simulink model "Duke_Simulink_13a"  (R2013a)
settings: Solver=FixedStepDiscrete  StartTime=0  StopTime=tempoSimulacao  FixedStep=1  RelTol=1e-3
values from neighbouring files (symbols this model uses):
  Ajustes_Inicial = dadosNumeroConstantes(linha)    [read_parametros_v2.m]
  aliquotaIR = dadosNumeroConstantes(linha)    [read_parametros_v2.m]
  CaixaInicial = dadosNumeroConstantes(linha)    [read_parametros_v2.m]
  Capital_Social_Inicial = CapitalSocial(1,2:end)    [Duke_main_v2.m]
  CFURH = dadosNumeroConstantes(linha)*TAR    [read_parametros_v2.m]
  contribuicaoCCEE = dadosNumeroConstantes(linha)    [read_parametros_v2.m]
  deducaoP_D = dadosNumeroConstantes(linha)    [read_parametros_v2.m]
  den_Ajustes = [1 zeros(1,PeriodoDepreciacao_Ajustes)]    [gera_Input_modelo.m]
  den_CustoAnual = [1 zeros(1,PeriodoCustoAnual-1)]    [gera_Input_modelo.m]
  den_CustoSemestral = [1 zeros(1,PeriodoCustoSemestral-1)]    [gera_Input_modelo.m]
  den_PPE_Edificacoes = [1 zeros(1,PPE_Periodo_Edificacoes)]    [gera_Input_modelo.m]
  den_PPE_Maquinas = [1 zeros(1,PPE_Periodo_Maquinas)]    [gera_Input_modelo.m]
  den_PPE_Moveis = [1 zeros(1,PPE_Periodo_Moveis)]    [gera_Input_modelo.m]
  den_PPE_Reservatorio = [1 zeros(1,PPE_Periodo_Reservatorio)]    [gera_Input_modelo.m]
  den_PPE_Veiculos = [1 zeros(1,PPE_Periodo_Veiculos)]    [gera_Input_modelo.m]
  DividaInicial = MtM_Total_Dividas(1,2:end)    [Duke_main_v2.m]
  Dividendos_A_Pagar_Inicial = dadosNumeroConstantes(linha)    [read_parametros_v2.m]
  garantiaFisica = dadosNumeroConstantes(linha)    [read_parametros_v2.m]
  IC_DividendosAPagarInicial = [repmat(vetor_DividendosAPagarInicial(1),numRealidades,1); zeros(realidadesPorSimulacao-numRealidades,1)]    [gera_Input_modelo.m]
  inicializa_JSCP = zeros(realidadesPorSimulacao,mes_JSCP)    [Duke_main_v2.m]
  IR_diferido_acumulado_inicial = dadosNumeroConstantes(linha)    [read_parametros_v2.m]
  JSCP_A_Pagar_Inicial = dadosNumeroConstantes(linha)    [read_parametros_v2.m]
  JSCP_ParcialPeriodo = dadosNumeroConstantes(linha)    [read_parametros_v2.m]
  JSCP_RetidoInicial = 0    [Duke_main_v2.m]
  Limite_Reserva_Lucros = dadosNumeroConstantes(linha)    [read_parametros_v2.m]
  Limite_Reserva_Lucros_Capital = dadosNumeroConstantes(linha)    [read_parametros_v2.m]
  LucroParcialPeriodo = dadosNumeroConstantes(linha)    [read_parametros_v2.m]
  LucroRetidoInicial = dadosNumeroConstantes(linha)    [read_parametros_v2.m]
  mes_DataInicial = month(DataInicial)    [Duke_main_v2.m]
  mes_JSCP = dadosNumeroConstantes(linha)    [read_parametros_v2.m]
  num_Ajustes = [0 ones(1,PeriodoDepreciacao_Ajustes)]*(1/PeriodoDepreciacao_Ajustes)    [gera_Input_modelo.m]
  num_CustoAnual = ones(1,PeriodoCustoAnual)*(1/PeriodoCustoAnual)    [gera_Input_modelo.m]
  num_CustoSemestral = ones(1,PeriodoCustoSemestral)*(1/PeriodoCustoSemestral)    [gera_Input_modelo.m]
  num_PPE_Edificacoes = [0 ones(1,PPE_Periodo_Edificacoes)]*(1/PPE_Periodo_Edificacoes)    [gera_Input_modelo.m]
  num_PPE_Maquinas = [0 ones(1,PPE_Periodo_Maquinas)]*(1/PPE_Periodo_Maquinas)    [gera_Input_modelo.m]
  num_PPE_Moveis = [0 ones(1,PPE_Periodo_Moveis)]*(1/PPE_Periodo_Moveis)    [gera_Input_modelo.m]
  num_PPE_Reservatorio = [0 ones(1,PPE_Periodo_Reservatorio)]*(1/PPE_Periodo_Reservatorio)    [gera_Input_modelo.m]
  num_PPE_Veiculos = [0 ones(1,PPE_Periodo_Veiculos)]*(1/PPE_Periodo_Veiculos)    [gera_Input_modelo.m]
  Outros_Passivos = dadosNumeroConstantes(linha)    [read_parametros_v2.m]
  periodoDividendos = dadosNumeroConstantes(linha)    [read_parametros_v2.m]
  periodoDividendos_delay = periodoDividendos    [Duke_main_v2.m]
  PeriodoIR_diferido = 12    [Duke_main_v2.m]
  PeriodoJSCP = 12    [Duke_main_v2.m]
  PIS_COFINS_Cumulativo = PIS + COFINS    [read_parametros_v2.m]
  PPE_Inicial_Edificacoes = dadosNumeroConstantes(linha)    [read_parametros_v2.m]
  PPE_Inicial_Maquinas = dadosNumeroConstantes(linha)    [read_parametros_v2.m]
  PPE_Inicial_Moveis = dadosNumeroConstantes(linha)    [read_parametros_v2.m]
  PPE_Inicial_Reservatorio = dadosNumeroConstantes(linha)    [read_parametros_v2.m]
  PPE_Inicial_Terreno = dadosNumeroConstantes(linha)    [read_parametros_v2.m]
  PPE_Inicial_Veiculos = dadosNumeroConstantes(linha)    [read_parametros_v2.m]
  refInd = (1-TEIFref)*(1-TEIPref)    [read_parametros_v2.m]
  Reserva_Capital_Inicial = dadosNumeroConstantes(linha)    [read_parametros_v2.m]
  Reserva_Lucros_Inicial = dadosNumeroConstantes(linha)    [read_parametros_v2.m]
  Taxa_Anual_Reserva = dadosNumeroConstantes(linha)    [read_parametros_v2.m]
  Taxa_diferimento = dadosNumeroConstantes(linha)    [read_parametros_v2.m]
  taxaMinorityInterest = dadosNumeroConstantes(linha)    [read_parametros_v2.m]
  TEIFa = dadosNumeroConstantes(linha)    [read_parametros_v2.m]
  TEIP = dadosNumeroConstantes(linha)    [read_parametros_v2.m]
  tempoSimulacao = 180    [Duke_main_v2.m]
  TEO = dadosNumeroConstantes(linha)    [read_parametros_v2.m]
  vetor_DividendosAPagarInicial = [repmat(vetor_DividendosAPagarInicial,numRealidades,1); zeros(realidadesPorSimulacao-numRealidades,periodoDividendos)]    [gera_Input_modelo.m]
  vetor_JSCP_APagarInicial = [repmat(vetor_JSCP_APagarInicial,numRealidades,1); zeros(realidadesPorSimulacao-numRealidades,PeriodoJSCP)]    [gera_Input_modelo.m]
undefined symbols (not defined in the file or in its folder): aDeducaoICMS, DiaPgtDespesasAdm, DiscIntNeverNeededParam, dts, IC_JSCP_APagarInicial, juros_ContasAPagar, juros_ContasAReceber, Media_DeprPPE, mediaADeducaoICMS, mediaADeducaoPISCOFINS, mediaRuidoGeracao, mediaTEIFa, mediaTEIP, Parametros, Periodo_Mes, PPE_Inicial, r, ruidoGeracaoSeed, Seed_DeprPPE, seedADeducaoICMS, seedADeducaoPISCOFINS, TEIFaSeed, TEIPSeed, Var_DeprPPE, varianciaADeducaoICMS, varianciaADeducaoPISCOFINS, varianciaRuidoGeracao, varianciaTEIFa, varianciaTEIP
libraries: simulink x22, dspsrcs4 x12
(part 1 of 2)
settings Model: TunableVars=Ajustes_Inicial,CFURH,CaixaInicial,Capital_Social_Inicial,DividaInicial,IC_DividendosAPagarInicial,IR_diferido_acumulado_inicial,JSCP_ParcialPeriodo,JSCP_RetidoInicial,Limite_Reserva_Lucros,Limite_Reserva_Lucros_Capital,LucroParcialPeriodo,LucroRetidoInicial,Outros_Passivos,PIS_COFINS_Cumulativo,PPE_Inicial_Edificacoes,PPE_Inicial_Maquinas,PPE_Inicial_Moveis,PPE_Inicial_Reservatorio,PPE_Inicial_Terreno,PPE_Inicial_Veiculos,PeriodoIR_diferido,PeriodoJSCP,Reserva_Capital_Inicial,Reserva_Lucros_Inicial,TEIFa,TEIP,TEO,TFSEE,Taxa_Anual_Reserva,Taxa_diferimento,aliquotaIR,contribuicaoCCEE,deducaoP_D,den_Ajustes,den_PPE_Edificacoes,den_PPE_Maquinas,den_PPE_Moveis,den_PPE_Reservatorio,den_PPE_Veiculos,den_Premio,garantiaFisica,inicializa_JSCP,mes_DataInicial,mes_JSCP,num_Ajustes,num_PPE_Edificacoes,num_PPE_Maquinas,num_PPE_Moveis,num_PPE_Reservatorio,num_PPE_Veiculos,num_Premio,periodoDividendos,periodoDividendos_delay,refInd,taxaMinorityInterest,vetor_DividendosAPagarInicial,vetor_JSCP_APagarInicial  TunableVarsStorageClass=Auto,Auto,Auto,Auto,Auto,Auto,Auto,Auto,Auto,Auto,Auto,Auto,Auto,Auto,Auto,Auto,Auto,Auto,Auto,Auto,Auto,Auto,Auto,Auto,Auto,Auto,Auto,Auto,Auto,Auto,Auto,Auto,Auto,Auto,Auto,Auto,Auto,Auto,Auto,Auto,Auto,Auto,Auto,Auto,Auto,Auto,Auto,Auto,Auto,Auto,Auto,Auto,Auto,Auto,Auto,Auto,Auto,Auto  TunableVarsTypeQualifier=,,,,,,,,,,,,,,,,,,,,,,,,,,,,,,,,,,,,,,,,,,,,,,,,,,,,,,,,,  Creator=sergio.junior  LastModifiedBy=Felipe
settings DataIOCC: ExternalInput=Input  LoadExternalInput=on  SaveFormat=StructureWithTime
settings OptimizationCC: InlineParams=on  ExpressionDepthLimit=2147483647
settings DebuggingCC: MultiTaskDSMMsg=warning  MultiTaskCondExecSysMsg=none  MultiTaskRateTransMsg=warning
settings HardwareCC: TargetIntDivRoundTo=Zero  TargetEndianess=LittleEndian  TargetHWDeviceType=MATLAB Host  ProdEqTarget=off
settings SFSimCC: SimParseCustomCode=off
settings RTWCC: SystemTargetFile=rsim.tlc  TemplateMakefile=rsim_default_tmf  Description=Rapid Simulation Target  ProcessScript=rsim_make_rtw_hook  IncludeERTFirstTime=on  RTWCompilerOptimization=On
settings RSimTargetCC: CodeReplacementLibrary=C89/C90 (ANSI)  ERTMultiwordTypeDef=System defined  ERTMultiwordLength=256  IsPILTarget=off  LogVarNameModifier=none  EnableShiftOperators=on  RSIM_SOLVER_SELECTION=UseSolverModule

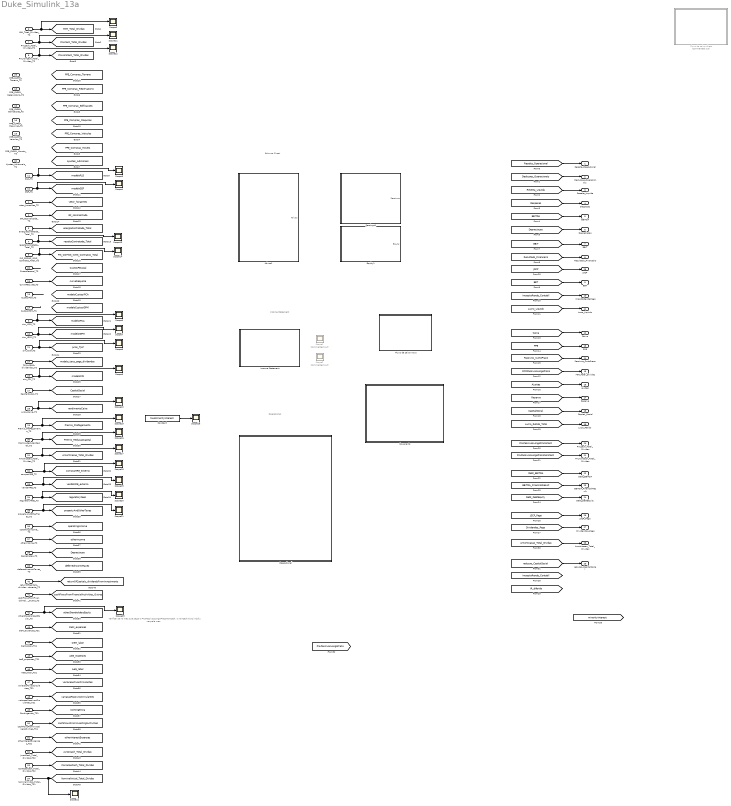
== system Duke_Simulink_13a ==
  note: Operacional
  note: Income Statement
  note: Balance Sheet
  note: Verificar se no mes que paga o PnLPassivosLongoPrazoNonCash, o nonCash é oq incidiu naquele mes
  vetor_horasMes_TS : Inport
  GF_sazonalizada_TS : Inport  Port=2
  energiaContratada_Total_TS : Inport  Port=3
  receitaContratada_Total_TS : Inport  Port=4  PortDimensions=realidadesPorSimulacao
  PIS_COFINS_ICMS_Contratos_Total_TS : Inport  Port=5  PortDimensions=realidadesPorSimulacao
  MtM_Total_Dividas_TS : Inport  Port=6  PortDimensions=realidadesPorSimulacao
  PnLCash_Total_Dividas_TS : Inport  Port=7  PortDimensions=realidadesPorSimulacao
  PnLnonCash_Total_Dividas_TS : Inport  Port=8  PortDimensions=realidadesPorSimulacao
  sim_IPCA_TS : Inport  Port=9  PortDimensions=realidadesPorSimulacao
  sim_IGPM_TS : Inport  Port=10  PortDimensions=realidadesPorSimulacao
  PLD_TS : Inport  Port=11  PortDimensions=realidadesPorSimulacao
  GSF_TS : Inport  Port=12  PortDimensions=realidadesPorSimulacao
  CustosIPCA_TS : Inport  Port=13
  CustosIGPM_TS : Inport  Port=14
  PPE_CAPEX_Edificacoes_TS : Inport  Port=15
  PPE_CAPEX_Maquinas_TS : Inport  Port=16
  PPE_CAPEX_Moveis_TS : Inport  Port=17
  PPE_CAPEX_Reservatorio_TS : Inport  Port=18
  PPE_CAPEX_Veiculos_TS : Inport  Port=19
  Ajustes_Adicionais_TS : Inport  Port=20
  sim_TJLP_TS : Inport  Port=21  PortDimensions=realidadesPorSimulacao
  CustosPessoal_TS : Inport  Port=22
  CurvaReajuste_TS : Inport  Port=23
  taxa_paga_dividendos_TS : Inport  Port=24
  sim_CDI_TS : Inport  Port=25  PortDimensions=realidadesPorSimulacao
  PPE_CAPEX_Terreno_TS : Inport  Port=26
  CapitalSocial_TS : Inport  Port=27
  juros_Caixa_TS : Inport  Port=28  PortDimensions=realidadesPorSimulacao
  Premio_PrePagamento_TS : Inport  Port=29  PortDimensions=realidadesPorSimulacao
  Premio_ReducaoCapital_TS : Inport  Port=30  PortDimensions=realidadesPorSimulacao
  Amortizacao_Total_Dividas_TS : Inport  Port=31  PortDimensions=realidadesPorSimulacao
  compraMRE_TS : Inport  Port=32
  vendaMRE_TS : Inport  Port=33
  regulatoryFees_TS : Inport  Port=34
  propertyAndOtherTaxes_TS : Inport  Port=35
  operatingIncome_TS : Inport  Port=36
  otherIncome_TS : Inport  Port=37
  depreciacao_TS : Inport  Port=38
  deferredIncomeTaxes_TS : Inport  Port=39
  returnOfCapitals_dividendsFromInvestments_TS : Inport  Port=40
  cashFlowsFromFinancialActivities_Outros_TS : Inport  Port=41
  otherShareholdersEquity_TS : Inport  Port=42
  OeM_expenses_TS1 : Inport  Port=43
  OeM_labor_TS1 : Inport  Port=44
  AeG_expenses_TS1 : Inport  Port=45
  AeG_labor_TS1 : Inport  Port=46
  variacaoAtivosCirculantes_TS1 : Inport  Port=47
  variacaoPassivosCirculantes_TS1 : Inport  Port=48
  Contingencia_TS1 : Inport  Port=49
  cashFlowsFromInvestinglActivities_TS1 : Inport  Port=50
  otherInterestExpenses_TS2 : Inport  Port=51
  JurosCash_Total_Dividas_TS2 : Inport  Port=52  PortDimensions=realidadesPorSimulacao
  CorrecaoCash_Total_Dividas_TS2 : Inport  Port=53  PortDimensions=realidadesPorSimulacao
  NominalInicial_Total_Dividas_TS1 : Inport  Port=54
  Ativos1 : Subsystem
  Constant : Constant  Value=taxaMinorityInterest
  Covenants : Subsystem
  Equity1 : Subsystem
  Fluxo de caixa direto : Subsystem  Commented=on
  Fluxo de caixa novo : Subsystem
  Income Statement : Subsystem
  Operacional : Subsystem
  Passivos1 : Subsystem
  Scope1 : Scope  Commented=on
      settings: TimeRange=500  YMin=-50000  YMax=450000  SaveName=ScopeData10
  Scope{3..22,25..26} (22 alike) : Scope
      Scope10 settings: YMin=0  YMax=65000  SaveName=ScopeData132
      Scope11 settings: YMin=0  YMax=65000  SaveName=ScopeData133
      Scope12 settings: YMin=0  YMax=65000  SaveName=ScopeData134
      Scope13 settings: YMin=0  YMax=65000  SaveName=ScopeData135
      Scope14 settings: YMin=0  YMax=65000  SaveName=ScopeData136
      Scope15 settings: YMin=0  YMax=65000  SaveName=ScopeData163
      Scope16 settings: YMin=0  YMax=65000  SaveName=ScopeData164
      Scope17 settings: YMin=0  YMax=65000  SaveName=ScopeData167
      Scope18 settings: YMin=0  YMax=65000  SaveName=ScopeData169
      Scope19 settings: YMin=0  YMax=65000  SaveName=ScopeData170
      Scope20 settings: YMin=0  YMax=65000  SaveName=ScopeData171
      Scope21 settings: YMin=0  YMax=65000  SaveName=ScopeData172
      Scope22 settings: YMin=0  YMax=65000  SaveName=ScopeData89
      Scope25 settings: YMin=0  YMax=65000  SaveName=ScopeData176
      Scope26 settings: YMin=0  YMax=65000  SaveName=ScopeData177
      Scope3 settings: YMin=0  YMax=65000  SaveName=ScopeData126
      Scope4 settings: YMin=0  YMax=65000  SaveName=ScopeData127
      Scope5 settings: YMin=0  YMax=65000  SaveName=ScopeData128
      Scope6 settings: YMin=0  YMax=65000  SaveName=ScopeData118
      Scope7 settings: YMin=0  YMax=65000  SaveName=ScopeData129
      Scope8 settings: YMin=0  YMax=65000  SaveName=ScopeData130
      Scope9 settings: YMin=0  YMax=65000  SaveName=ScopeData131
  Scope2 : Scope  Commented=on
      settings: TimeRange=500  YMin=-50000  YMax=450000  SaveName=ScopeData11
  Receita_Operacional : Outport
  Deducoes_Operacionais : Outport  Port=2
  Receita_Liquida : Outport  Port=3
  Despesas : Outport  Port=4
  EBITDA : Outport  Port=5
  Depreciacao : Outport  Port=6
  EBIT : Outport  Port=7
  Resultado_Financeiro : Outport  Port=8
  EBT : Outport  Port=9
  ImpostoRendaPago : Outport  Port=10
  Lucro_Liquido : Outport  Port=11
  Caixa : Outport  Port=12
  PPE : Outport  Port=13
  Passivos_CurtoPrazo : Outport  Port=14
  MtM_Total_Dividas : Outport  Port=15
  Ajustes : Outport  Port=16
  Reserva : Outport  Port=17
  Capital_Social : Outport  Port=18
  Lucro_Retido : Outport  Port=19
  PnLCash_Total_Dividas : Outport  Port=20
  PnLnonCash_Total_Dividas : Outport  Port=21
  Debt_EBITDA : Outport  Port=22
  EBITDA_FinancialResult : Outport  Port=23
  Debt_DebtEquity : Outport  Port=24
  JSCP : Outport  Port=25
  JSCP_Pago : Outport  Port=26
  Dividendos_Pago : Outport  Port=27
  Amortizacao_Total_Dividas : Outport  Port=28
  reducao_CapitalSocial : Outport  Port=29
  tag scope: AeG_expenses=global, AeG_labor=global, Ajustes_Adicionais=global, Amortizacao_Total_Dividas=global, CapitalSocial=global, Contingencia=global, CorrecaoCash_Total_Dividas=global, CustosPessoal=global, Depreciacao=global, GF_sazonalizada=global, JurosCash_Total_Dividas=global, MtM_Total_Dividas=global, NominalInicial_Total_Dividas=global, OeM_expenses=global, OeM_labor=global, PIS_COFINS_ICMS_Contratos_Total=global, PPE_Compras_Edificacoes=global, PPE_Compras_Maquinas=global, PPE_Compras_Moveis=global, PPE_Compras_Reservatorio=global, PPE_Compras_Terreno=global, PPE_Compras_Veiculos=global, PnLCash_Total_Dividas=global, PnLnonCash_Total_Dividas=global, Premio_PrePagamento=global, Premio_ReducaoCapital=global, cashFlowsFromFinancialActivities_Outros=global, cashFlowsFromInvestinglActivities=global, compraMRE_externo=global, curvaReajuste=global, deferredIncomeTaxes=global, energiaContratada_Total=global, juros_TJLP=global, modeloCDI=global, modeloCustosIGPM=global, modeloCustosIPCA=global, modeloGSF=global, modeloIGPM=global, modeloIPCA=global, modeloPLD=global, modelo_taxa_paga_dividendos=global, operatingIncome=global, otherIncome=global, otherInterestExpenses=global, otherShareholdersEquity=global, propertyAndOtherTaxes=global, receitaContratada_Total=global, regulatoryFees=global, rendimentoCaixa=global, returnOfCapitals_dividendsFromInvestments=global, variacaoAtivosCirculantes=global, variacaoPassivosCirculantes=global, vendaMRE_externo=global, vetor_horasMes=global
  wires:
  [Receita_Operacional] -> Receita_Operacional/1
  [Deducoes_Operacionais] -> Deducoes_Operacionais/1
  [Receita_Liquida] -> Receita_Liquida/1
  [Despesas] -> Despesas/1
  [EBITDA] -> EBITDA/1
  [Depreciacao] -> Depreciacao/1
  [EBIT] -> EBIT/1
  [Resultado_Financeiro] -> Resultado_Financeiro/1
  [EBT] -> EBT/1
  [ImpostoRenda_Contabil] -> ImpostoRendaPago/1
  [Lucro_Liquido] -> Lucro_Liquido/1
  [Caixa] -> Caixa/1
  [PPE] -> PPE/1
  [Passivos_CurtoPrazo] -> Passivos_CurtoPrazo/1
  [MtMPassivosLongoPrazo] -> MtM_Total_Dividas/1
  [Ajustes] -> Ajustes/1
  [Reserva] -> Reserva/1
  [CapitalSocial] -> Capital_Social/1
  [Lucro_Retido_Total] -> Lucro_Retido/1
  [PnLPassivosLongoPrazoCash] -> PnLCash_Total_Dividas/1
  [PnLPassivosLongoPrazoNonCash] -> PnLnonCash_Total_Dividas/1
  [Debt_EBITDA] -> Debt_EBITDA/1
  [EBITDA_FinancialResult] -> EBITDA_FinancialResult/1
  [Debt_DebtEquity] -> Debt_DebtEquity/1
  MtM_Total_Dividas_TS/1 -> Scope6/1, [MtM_Total_Dividas]
  PnLCash_Total_Dividas_TS/1 -> Scope11/1, [PnLCash_Total_Dividas]
  PnLnonCash_Total_Dividas_TS/1 -> Scope12/1, [PnLnonCash_Total_Dividas]
  ? -> [PPE_Compras_Reservatorio]
  ? -> [PPE_Compras_Edificacoes]
  ? -> [PPE_Compras_Maquinas]
  ? -> [PPE_Compras_Veiculos]
  ? -> [PPE_Compras_Moveis]
  ? -> [Ajustes_Adicionais]
  PLD_TS/1 -> Scope3/1, [modeloPLD]
  GSF_TS/1 -> Scope4/1, [modeloGSF]
  vetor_horasMes_TS/1 -> [vetor_horasMes]
  GF_sazonalizada_TS/1 -> [GF_sazonalizada]
  energiaContratada_Total_TS/1 -> [energiaContratada_Total]
  receitaContratada_Total_TS/1 -> Scope13/1, [receitaContratada_Total]
  PIS_COFINS_ICMS_Contratos_Total_TS/1 -> Scope14/1, [PIS_COFINS_ICMS_Contratos_Total]
  CustosPessoal_TS/1 -> ?
  CurvaReajuste_TS/1 -> [curvaReajuste]
  CustosIPCA_TS/1 -> ?
  CustosIGPM_TS/1 -> ?
  sim_IPCA_TS/1 -> Scope5/1, [modeloIPCA]
  sim_IGPM_TS/1 -> Scope7/1, [modeloIGPM]
  sim_TJLP_TS/1 -> Scope8/1, [juros_TJLP]
  [JSCP] -> JSCP/1
  taxa_paga_dividendos_TS/1 -> [modelo_taxa_paga_dividendos]
  sim_CDI_TS/1 -> Scope9/1, [modeloCDI]
  ? -> [PPE_Compras_Terreno]
  CapitalSocial_TS/1 -> [CapitalSocial]
  juros_Caixa_TS/1 -> Scope10/1, [rendimentoCaixa]
  [JSCP_Pago] -> JSCP_Pago/1
  [Dividendos_Pago] -> Dividendos_Pago/1
  Premio_PrePagamento_TS/1 -> [Premio_PrePagamento], Scope15/1
  Premio_ReducaoCapital_TS/1 -> [Premio_ReducaoCapital], Scope16/1
  Amortizacao_Total_Dividas_TS/1 -> Scope17/1, [Amortizacao_Total_Dividas]
  [Amortizacao_Total_Dividas] -> Amortizacao_Total_Dividas/1
  [reducao_CapitalSocial] -> reducao_CapitalSocial/1
  compraMRE_TS/1 -> Scope18/1, [compraMRE_externo]
  vendaMRE_TS/1 -> Scope19/1, [vendaMRE_externo]
  regulatoryFees_TS/1 -> Scope20/1, [regulatoryFees]
  propertyAndOtherTaxes_TS/1 -> Scope21/1, [propertyAndOtherTaxes]
  operatingIncome_TS/1 -> [operatingIncome]
  otherIncome_TS/1 -> [otherIncome]
  depreciacao_TS/1 -> [Depreciacao]
  deferredIncomeTaxes_TS/1 -> [deferredIncomeTaxes]
  returnOfCapitals_dividendsFromInvestments_TS/1 -> [returnOfCapitals_dividendsFromInvestments]
  cashFlowsFromFinancialActivities_Outros_TS/1 -> [cashFlowsFromFinancialActivities_Outros]
  otherShareholdersEquity_TS/1 -> Scope25/1, [otherShareholdersEquity]
  Constant/1 -> Scope26/1
  OeM_expenses_TS1/1 -> [OeM_expenses]
  OeM_labor_TS1/1 -> [OeM_labor]
  AeG_expenses_TS1/1 -> [AeG_expenses]
  AeG_labor_TS1/1 -> [AeG_labor]
  variacaoAtivosCirculantes_TS1/1 -> [variacaoAtivosCirculantes]
  variacaoPassivosCirculantes_TS1/1 -> [variacaoPassivosCirculantes]
  Contingencia_TS1/1 -> [Contingencia]
  cashFlowsFromInvestinglActivities_TS1/1 -> [cashFlowsFromInvestinglActivities]
  otherInterestExpenses_TS2/1 -> [otherInterestExpenses]
  JurosCash_Total_Dividas_TS2/1 -> [JurosCash_Total_Dividas]
  CorrecaoCash_Total_Dividas_TS2/1 -> [CorrecaoCash_Total_Dividas]
  NominalInicial_Total_Dividas_TS1/1 -> Scope22/1, [NominalInicial_Total_Dividas]

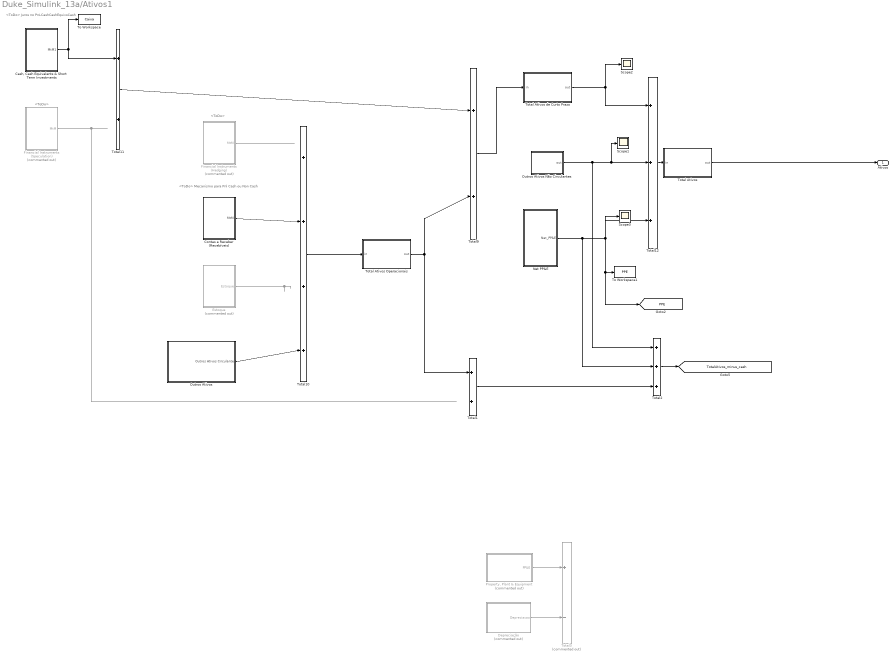
== system Duke_Simulink_13a/Ativos1 ==
  note: <ToDo>
      | Mecanismo para
      | Pnl Cash ou Non Cash
  note: <ToDo>
  note: <ToDo>
      | Juros no
      | PnLCashCashEquivsCash
  note: <ToDo>
  "Cash, Cash Equivalents & Short Term Investments" : Subsystem
  Contas a Receber (Recebíveis) : Subsystem
  Depreciação : Subsystem  Commented=on
  Estoque : Subsystem  Commented=on
  Financial Instruments (Hedging) : Subsystem  Commented=on
  Financial Instruments (Speculation) : Subsystem  Commented=on
  Net PP&E : Subsystem
  Outros Ativos : Subsystem
  Outros Ativos Não Circulantes : Subsystem
  "Property, Plant & Equipment" : Subsystem  Commented=on
  Scope1 : Scope
      settings: SaveName=ScopeData73
  Scope2 : Scope
      settings: SaveName=ScopeData74
  Scope3 : Scope
      settings: SaveName=ScopeData72
  To Workspace : ToWorkspace  VariableName=Caixa  SampleTime=-1  SaveFormat=Timeseries
  To Workspace1 : ToWorkspace  VariableName=PPE  SampleTime=-1  SaveFormat=Timeseries
  Total Ativos : Subsystem
  Total Ativos Operacionais : Subsystem
  Total Ativos de Curto Prazo : Subsystem
  Total1 : Sum
  Total10 : Sum  Inputs=+|+|+|+
  Total11 : Sum  Inputs=+|+
  Total12 : Sum  Inputs=+||+||+
  Total2 : Sum  Inputs=+++
  Total3 : Sum  Commented=on  Inputs=+-
  Total9 : Sum  Inputs=+||+
  "Ativos    " : Outport
  tag scope: PPE=global, TotalAtivos_minus_cash=global
  wires:
  Estoque/1(Estoque) -> ?
  Financial Instruments (Speculation)/1(MtM) -> ?
  Financial Instruments (Hedging)/1(MtM) -> ?
  Total11/1 -> Total9/1
  Total10/1 -> Total Ativos Operacionais/1(in)
  Total Ativos Operacionais/1(out) -> Total9/2, Total1/1
  Total9/1 -> Total Ativos de Curto Prazo/1(in)
  Total12/1 -> Total Ativos/1(in)
  Total Ativos de Curto Prazo/1(out) -> Scope2/1, Total12/1
  "Cash, Cash Equivalents & Short Term Investments"/1(MtM1) -> To Workspace/1, Total11/1
  Total1/1 -> Total2/3
  Total2/1 -> [TotalAtivos_minus_cash]
  "Property, Plant & Equipment"/1(PP&E) -> Total3/1
  Outros Ativos Não Circulantes/1(out) -> Total2/1, Scope1/1, Total12/2
  Net PP&E/1(Net_PP&E) -> Total2/2, Total12/3, Scope3/1, To Workspace1/1, [PPE]
  Depreciação/1(Depreciacao) -> Total3/2
  Outros Ativos/1(Outros Ativos Circulantes) -> Total10/4
  Contas a Receber (Recebíveis)/1(MtM) -> Total10/2
  Total Ativos/1(out) -> "Ativos    "/1

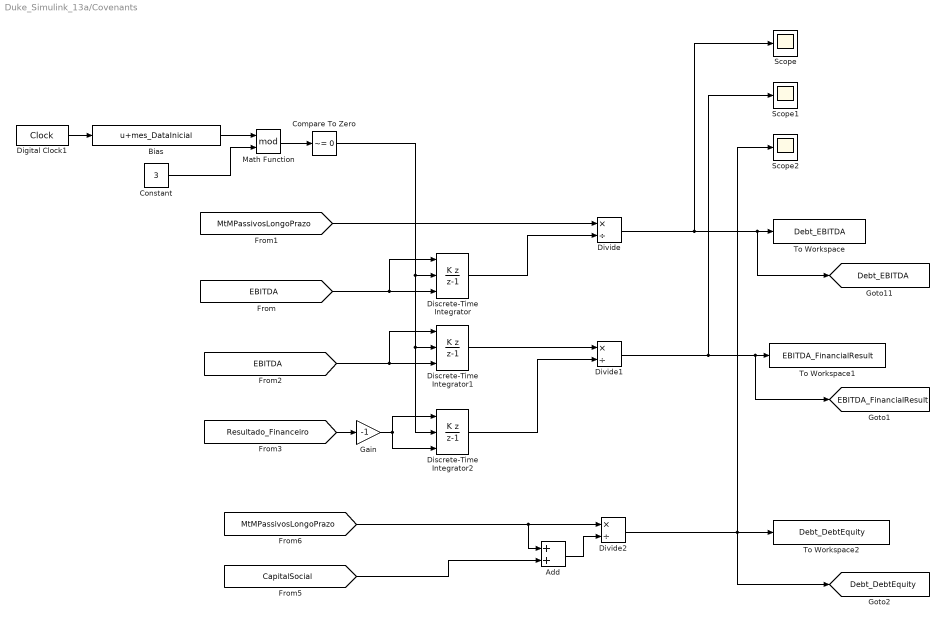
== system Duke_Simulink_13a/Covenants ==
  Add : Sum
  Bias : Bias  Bias=mes_DataInicial
  Compare To Zero : simulink/Logic and Bit Operations/Compare To Zero  relop=~=  OutDataTypeStr=boolean
  Constant : Constant  Value=3
  Digital Clock1 : DigitalClock
  Discrete-Time Integrator : DiscreteIntegrator  IntegratorMethod=Accumulation: Backward Euler  ExternalReset=rising  InitialConditionSource=external  ICPrevOutput=DiscIntNeverNeededParam  ICPrevScaledInput=DiscIntNeverNeededParam
  Discrete-Time Integrator1 : DiscreteIntegrator  IntegratorMethod=Accumulation: Backward Euler  ExternalReset=rising  InitialConditionSource=external  ICPrevOutput=DiscIntNeverNeededParam  ICPrevScaledInput=DiscIntNeverNeededParam
  Discrete-Time Integrator2 : DiscreteIntegrator  IntegratorMethod=Accumulation: Backward Euler  ExternalReset=rising  InitialConditionSource=external  ICPrevOutput=DiscIntNeverNeededParam  ICPrevScaledInput=DiscIntNeverNeededParam
  Divide : Product  Inputs=*/  SampleTime=1
  Divide1 : Product  Inputs=*/  SampleTime=1
  Divide2 : Product  Inputs=*/  SampleTime=1
  Gain : Gain  Gain=-1
  Math Function : Math  Operator=mod  SaturateOnIntegerOverflow=on
  Scope : Scope
      settings: SaveName=ScopeData47
  Scope1 : Scope
      settings: SaveName=ScopeData48
  Scope2 : Scope
      settings: SaveName=ScopeData49
  To Workspace : ToWorkspace  VariableName=Debt_EBITDA  SampleTime=1  SaveFormat=Timeseries
  To Workspace1 : ToWorkspace  VariableName=EBITDA_FinancialResult  SampleTime=1  SaveFormat=Timeseries
  To Workspace2 : ToWorkspace  VariableName=Debt_DebtEquity  SampleTime=1  SaveFormat=Timeseries
  tag scope: Debt_DebtEquity=global, Debt_EBITDA=global, EBITDA_FinancialResult=global
  wires:
  [EBITDA] -> Discrete-Time Integrator/1, Discrete-Time Integrator/3
  Divide/1 -> [Debt_EBITDA], To Workspace/1, Scope/1
  Divide1/1 -> Scope1/1, [EBITDA_FinancialResult], To Workspace1/1
  Divide2/1 -> [Debt_DebtEquity], Scope2/1, To Workspace2/1
  Constant/1 -> Math Function/2
  Math Function/1 -> Compare To Zero/1
  Compare To Zero/1 -> Discrete-Time Integrator2/2, Discrete-Time Integrator1/2, Discrete-Time Integrator/2
  [EBITDA] -> Discrete-Time Integrator1/1, Discrete-Time Integrator1/3
  [Resultado_Financeiro] -> Gain/1
  [MtMPassivosLongoPrazo] -> Divide/1
  Discrete-Time Integrator/1 -> Divide/2
  Discrete-Time Integrator1/1 -> Divide1/1
  Discrete-Time Integrator2/1 -> Divide1/2
  [MtMPassivosLongoPrazo] -> Add/1, Divide2/1
  Gain/1 -> Discrete-Time Integrator2/1, Discrete-Time Integrator2/3
  Add/1 -> Divide2/2
  [CapitalSocial] -> Add/2
  Digital Clock1/1 -> Bias/1
  Bias/1 -> Math Function/1

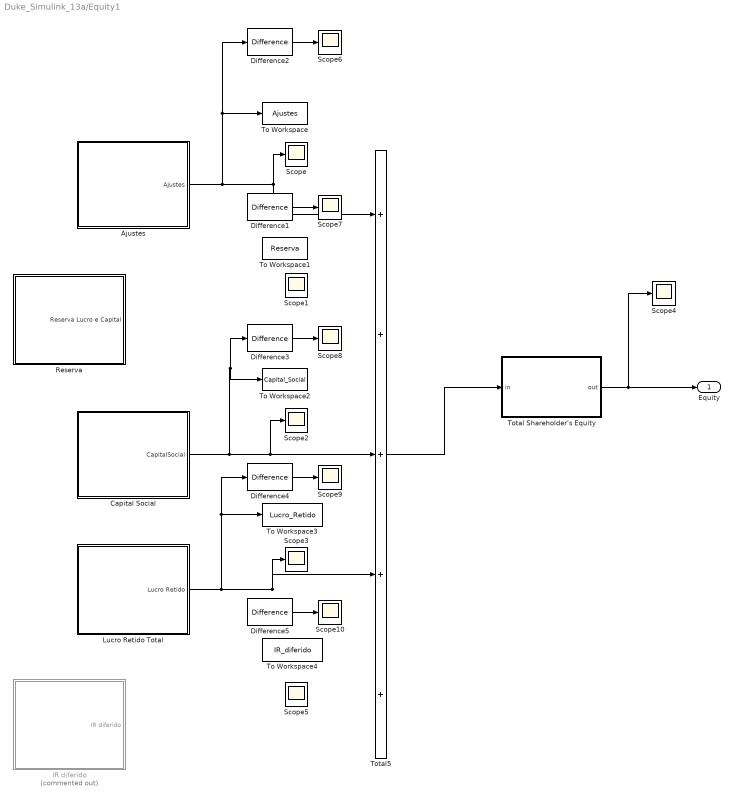
== system Duke_Simulink_13a/Equity1 ==
  Ajustes : Subsystem
  Capital Social : Subsystem
  Difference{1..5} (5 alike) : simulink/Discrete/Difference  ICPrevInput=0  InputProcessing=Inherited  OutMin=[]  OutMax=[]  OutDataType=fixdt(1, 16)  OutScaling=2^-10  DoSatur=off
  IR diferido : Subsystem  Commented=on
  Lucro Retido Total : Subsystem
  Reserva : Subsystem
  Scope{,1..10} (11 alike) : Scope
      Scope settings: SaveName=ScopeData81
      Scope1 settings: SaveName=ScopeData82
      Scope10 settings: SaveName=ScopeData153
      Scope2 settings: SaveName=ScopeData83
      Scope3 settings: SaveName=ScopeData84
      Scope4 settings: SaveName=ScopeData36
      Scope5 settings: SaveName=ScopeData119
      Scope6 settings: SaveName=ScopeData149
      Scope7 settings: SaveName=ScopeData150
      Scope8 settings: SaveName=ScopeData151
      Scope9 settings: SaveName=ScopeData152
  To Workspace : ToWorkspace  VariableName=Ajustes  SampleTime=-1  SaveFormat=Timeseries
  To Workspace1 : ToWorkspace  VariableName=Reserva  SampleTime=-1  SaveFormat=Timeseries
  To Workspace2 : ToWorkspace  VariableName=Capital_Social  SampleTime=-1  SaveFormat=Timeseries
  To Workspace3 : ToWorkspace  VariableName=Lucro_Retido  SampleTime=-1  SaveFormat=Timeseries
  To Workspace4 : ToWorkspace  VariableName=IR_diferido  SampleTime=-1  SaveFormat=Timeseries
  Total Shareholder's Equity : Subsystem
  Total5 : Sum  Inputs=+|+|+|+|+
  "Equity    " : Outport
  wires:
  Lucro Retido Total/1(Lucro Retido) -> Difference4/1, To Workspace3/1, Scope3/1, Total5/4
  Total5/1 -> Total Shareholder's Equity/1(in)
  Ajustes/1(Ajustes) -> Difference2/1, To Workspace/1, Scope/1, Total5/1
  ? -> Difference1/1, To Workspace1/1, Scope1/1, Total5/2
  Capital Social/1(CapitalSocial) -> Difference3/1, To Workspace2/1, Scope2/1, Total5/3
  Total Shareholder's Equity/1(out) -> Scope4/1, "Equity    "/1
  ? -> Total5/5, Scope5/1, Difference5/1, To Workspace4/1
  Difference2/1 -> Scope6/1
  Difference1/1 -> Scope7/1
  Difference3/1 -> Scope8/1
  Difference4/1 -> Scope9/1
  Difference5/1 -> Scope10/1

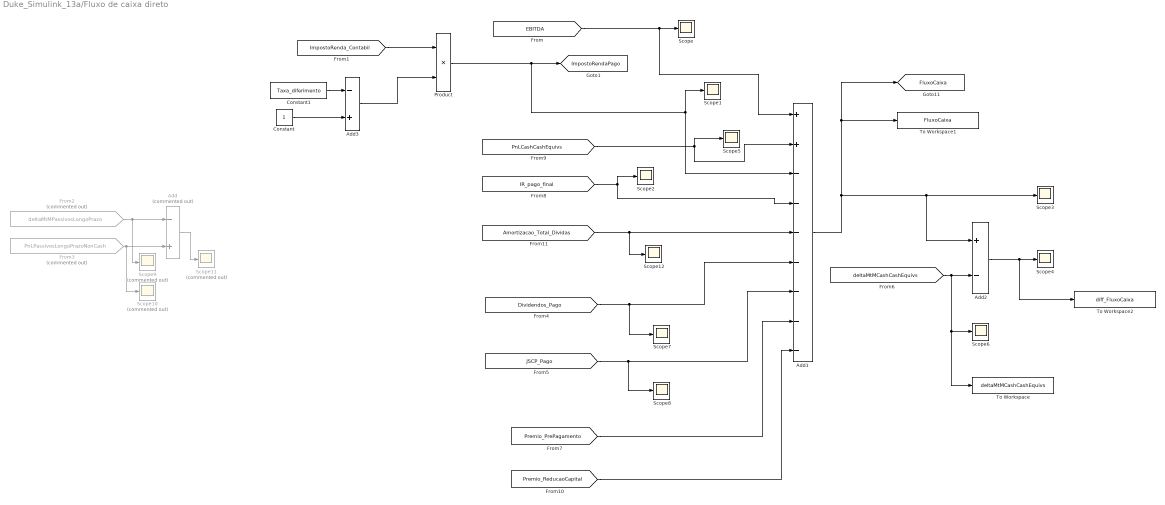
== system Duke_Simulink_13a/Fluxo de caixa direto ==
  Add : Sum  Commented=on  Inputs=-+
  Add1 : Sum  Inputs=++-------
  Add2 : Sum  Inputs=+-
  Add3 : Sum  Inputs=-+
  Constant : Constant
  Constant1 : Constant  Value=Taxa_diferimento
  From2 : From  Commented=on  GotoTag=deltaMtMPassivosLongoPrazo  TagVisibility=global
  From3 : From  Commented=on  GotoTag=PnLPassivosLongoPrazoNonCash  TagVisibility=global
  Product : Product
  Scope{,1..8,12} (10 alike) : Scope
      Scope settings: SaveName=ScopeData47
      Scope1 settings: SaveName=ScopeData48
      Scope12 settings: SaveName=ScopeData168
      Scope2 settings: SaveName=ScopeData53
      Scope3 settings: TimeRange=10  SaveName=ScopeData50
      Scope4 settings: TimeRange=450  YMin=-2e-06  YMax=2e-06  SaveName=ScopeData52
      Scope5 settings: SaveName=ScopeData125
      Scope6 settings: TimeRange=450  YMin=-15000000000  YMax=15000000000  SaveName=ScopeData66
      Scope7 settings: SaveName=ScopeData68
      Scope8 settings: SaveName=ScopeData69
  Scope10 : Scope  Commented=on
      settings: SaveName=ScopeData138
  Scope11 : Scope  Commented=on
      settings: SaveName=ScopeData139
  Scope9 : Scope  Commented=on
      settings: SaveName=ScopeData137
  To Workspace : ToWorkspace  VariableName=deltaMtMCashCashEquivs  SampleTime=-1  SaveFormat=Timeseries
  To Workspace1 : ToWorkspace  VariableName=FluxoCaixa  SampleTime=-1  SaveFormat=Timeseries
  To Workspace2 : ToWorkspace  VariableName=diff_FluxoCaixa  SampleTime=-1  SaveFormat=Timeseries
  tag scope: FluxoCaixa=global, ImpostoRendaPago=global
  wires:
  From2/1 -> Scope9/1, Add/1
  From3/1 -> Scope10/1, Add/2
  Add/1 -> Scope11/1
  Product/1 -> Add1/3, Scope1/1, [ImpostoRendaPago]
  Add2/1 -> To Workspace2/1, Scope4/1
  [deltaMtMCashCashEquivs] -> To Workspace/1, Scope6/1, Add2/2
  Add1/1 -> [FluxoCaixa], To Workspace1/1, Add2/1, Scope3/1
  [EBITDA] -> Add1/1, Scope/1
  [Dividendos_Pago] -> Add1/6, Scope7/1
  [JSCP_Pago] -> Add1/7, Scope8/1
  [ImpostoRenda_Contabil] -> Product/1
  Constant1/1 -> Add3/1
  Add3/1 -> Product/2
  Constant/1 -> Add3/2
  [IR_pago_final] -> Add1/4, Scope2/1
  [PnLCashCashEquivs] -> Scope5/1, Add1/2
  [Premio_PrePagamento] -> Add1/8
  [Premio_ReducaoCapital] -> Add1/9
  [Amortizacao_Total_Dividas] -> Scope12/1, Add1/5

== system Duke_Simulink_13a/Fluxo de caixa novo ==
  Add1 : Sum  Inputs=+-+++++++---+-+-
  Discrete-Time Integrator2 : DiscreteIntegrator  IntegratorMethod=Accumulation: Backward Euler  InitialCondition=CaixaInicial  ICPrevOutput=DiscIntNeverNeededParam  ICPrevScaledInput=DiscIntNeverNeededParam
  Scope3 : Scope
      settings: TimeRange=10  SaveName=ScopeData50
  Scope4 : Scope
      settings: TimeRange=450  YMin=-2e-06  YMax=2e-06  SaveName=ScopeData52
  tag scope: Caixa=global, cashFlow=global
  wires:
  [Lucro_Liquido] -> Add1/1
  [Depreciacao] -> Add1/2
  [minorityInterest] -> Add1/3
  [variacaoAtivosCirculantes] -> Add1/4
  [variacaoPassivosCirculantes] -> Add1/5
  [Contingencia] -> Add1/6
  [returnOfCapitals_dividendsFromInvestments] -> Add1/7
  [cashFlowsFromInvestinglActivities] -> Add1/8
  [cashFlowsFromFinancialActivities_Outros] -> Add1/9
  [JurosCash_Total_Dividas] -> Add1/11
  [CorrecaoCash_Total_Dividas] -> Add1/12
  [Amortizacao_Total_Dividas] -> Add1/10
  [NominalInicial_Total_Dividas] -> Add1/13
  ? -> Add1/14
  [PnLnonCash_Total_Dividas] -> Add1/15
  Add1/1 -> [cashFlow], Discrete-Time Integrator2/1
  Discrete-Time Integrator2/1 -> [Caixa]
  ? -> Add1/16

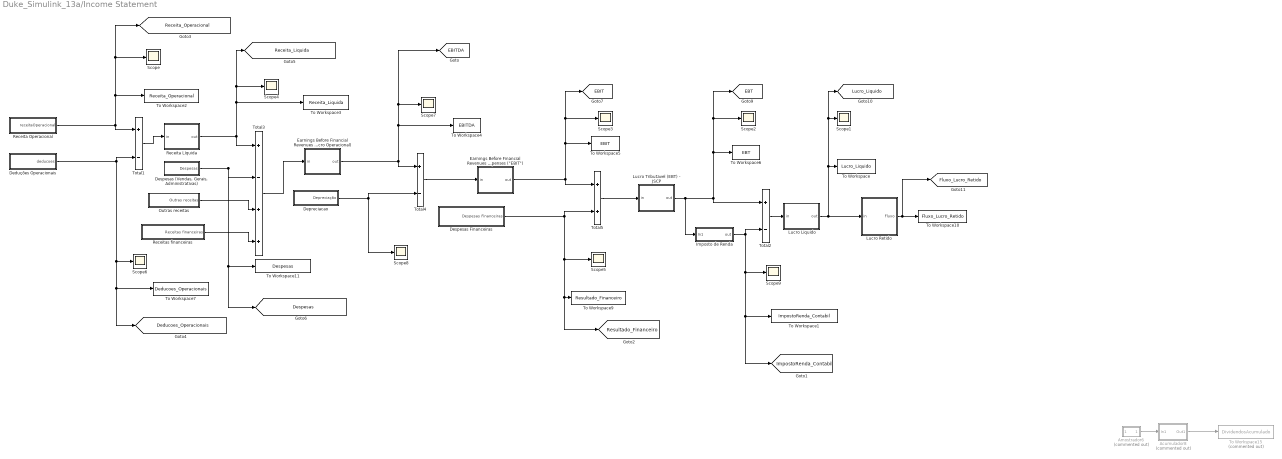
== system Duke_Simulink_13a/Income Statement ==
  Acumulador8 : Subsystem  Commented=on
  Amostrador6 : Subsystem  Commented=on
  Deduções Operacionais : Subsystem
  Depreciacao : Subsystem
  "Despesas (Vendas, Gerais, Administrativas)" : Subsystem
  Despesas Financeiras : Subsystem
  "Earnings Before Financial Revenues / Expenses, Depreciation and Amortization (\"EBITDA\") (Lucro Operacional)" : Subsystem
  "Earnings Before Financial Revenues and Expenses (\"EBIT\")" : Subsystem
  Imposto de Renda : Subsystem
  "Lucro Liquido " : Subsystem
  Lucro Retido : Subsystem
  Lucro Tributavel (EBT) - JSCP : Subsystem
  Outras receitas : Subsystem
  Receita Líquida : Subsystem
  Receita Operacional : Subsystem
  Receitas financeiras : Subsystem
  Scope{,1..9} (10 alike) : Scope
      Scope settings: SaveName=ScopeData5
      Scope1 settings: SaveName=ScopeData27
      Scope2 settings: SaveName=ScopeData28
      Scope3 settings: SaveName=ScopeData29
      Scope4 settings: SaveName=ScopeData8
      Scope5 settings: TimeRange=400  YMin=-15000000  YMax=0  SaveName=ScopeData31
      Scope6 settings: SaveName=ScopeData16
      Scope7 settings: SaveName=ScopeData15
      Scope8 settings: SaveName=ScopeData34
      Scope9 settings: SaveName=ScopeData46
  To Workspace : ToWorkspace  VariableName=Lucro_Liquido  SampleTime=-1  SaveFormat=Timeseries
  To Workspace1 : ToWorkspace  VariableName=ImpostoRenda_Contabil  SampleTime=-1  SaveFormat=Timeseries
  To Workspace10 : ToWorkspace  VariableName=Fluxo_Lucro_Retido  SampleTime=-1  SaveFormat=Timeseries
  To Workspace11 : ToWorkspace  VariableName=Despesas  SampleTime=-1  SaveFormat=Timeseries
  To Workspace15 : ToWorkspace  Commented=on  VariableName=DividendosAcumulado  SampleTime=-1  SaveFormat=Timeseries
  To Workspace2 : ToWorkspace  VariableName=Receita_Operacional  SampleTime=-1  SaveFormat=Timeseries
  To Workspace3 : ToWorkspace  VariableName=Receita_Liquida  SampleTime=-1  SaveFormat=Timeseries
  To Workspace4 : ToWorkspace  VariableName=EBITDA  SampleTime=-1  SaveFormat=Timeseries
  To Workspace5 : ToWorkspace  VariableName=EBIT  SampleTime=-1  SaveFormat=Timeseries
  To Workspace6 : ToWorkspace  VariableName=EBT  SampleTime=-1  SaveFormat=Timeseries
  To Workspace7 : ToWorkspace  VariableName=Deducoes_Operacionais  SampleTime=-1  SaveFormat=Timeseries
  To Workspace9 : ToWorkspace  VariableName=Resultado_Financeiro  SampleTime=-1  SaveFormat=Timeseries
  Total1 : Sum  Inputs=+|-
  Total2 : Sum  Inputs=+|-
  Total3 : Sum  Inputs=+|-|+|+
  Total4 : Sum  Inputs=+|-
  Total5 : Sum  Inputs=+|+
  tag scope: Deducoes_Operacionais=global, Despesas=global, EBIT=global, EBITDA=global, EBT=global, Fluxo_Lucro_Retido=global, ImpostoRenda_Contabil=global, Lucro_Liquido=global, Receita_Liquida=global, Receita_Operacional=global, Resultado_Financeiro=global
  wires:
  "Lucro Liquido "/1(out) -> Lucro Retido/1(in), [Lucro_Liquido], Scope1/1, To Workspace/1
  Acumulador8/1(Out1) -> To Workspace15/1
  Amostrador6/1(Out1) -> Acumulador8/1(In1)
  Receita Líquida/1(out) -> Total3/1, To Workspace3/1, [Receita_Liquida], Scope4/1
  "Earnings Before Financial Revenues / Expenses, Depreciation and Amortization (\"EBITDA\") (Lucro Operacional)"/1(out) -> [EBITDA], Scope7/1, To Workspace4/1, Total4/1
  Total4/1 -> "Earnings Before Financial Revenues and Expenses (\"EBIT\")"/1(in)
  "Earnings Before Financial Revenues and Expenses (\"EBIT\")"/1(out) -> To Workspace5/1, [EBIT], Scope3/1, Total5/1
  Total5/1 -> Lucro Tributavel (EBT) - JSCP/1(in)
  Lucro Tributavel (EBT) - JSCP/1(out) -> To Workspace6/1, [EBT], Scope2/1, Total2/1, Imposto de Renda/1(In1)
  Imposto de Renda/1(out) -> [ImpostoRenda_Contabil], To Workspace1/1, Scope9/1, Total2/2
  Total2/1 -> "Lucro Liquido "/1(in)
  Total1/1 -> Receita Líquida/1(in)
  Receita Operacional/1(receitaOperacional) -> To Workspace2/1, [Receita_Operacional], Scope/1, Total1/1
  Deduções Operacionais/1(deducoes) -> Scope6/1, [Deducoes_Operacionais], To Workspace7/1, Total1/2
  Depreciacao/1(Depreciação) -> Total4/2, Scope8/1
  Despesas Financeiras/1(Despesas Financeiras) -> [Resultado_Financeiro], To Workspace9/1, Scope5/1, Total5/2
  Lucro Retido/1(Fluxo) -> [Fluxo_Lucro_Retido], To Workspace10/1
  "Despesas (Vendas, Gerais, Administrativas)"/1(Despesas) -> Total3/2, [Despesas], To Workspace11/1
  Outras receitas/1(Outras receitas) -> Total3/3
  Receitas financeiras/1(Receitas financeiras) -> Total3/4
  Total3/1 -> "Earnings Before Financial Revenues / Expenses, Depreciation and Amortization (\"EBITDA\") (Lucro Operacional)"/1(in)

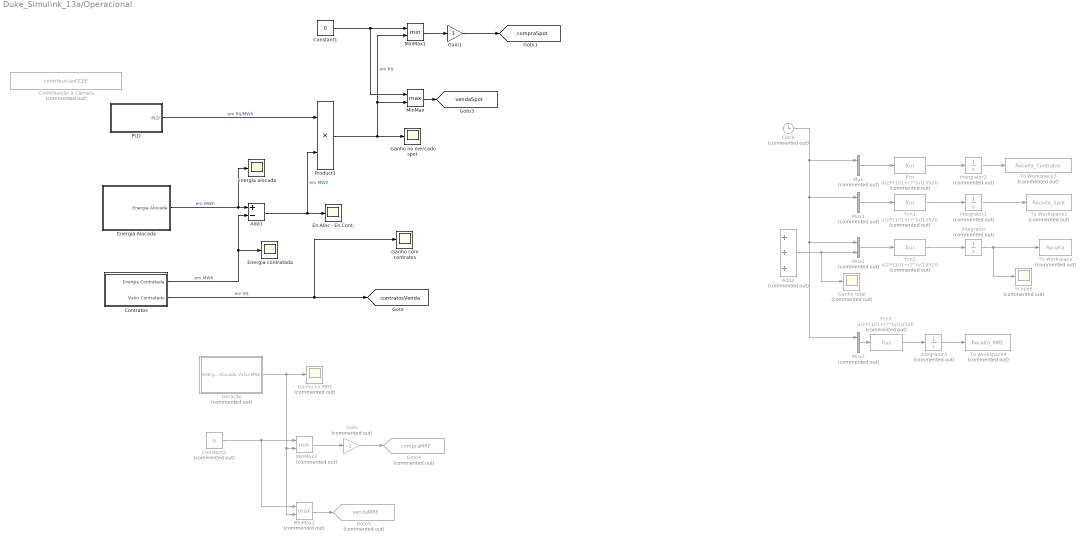
== system Duke_Simulink_13a/Operacional ==
  Add1 : Sum  Inputs=+-
  Add2 : Sum  Commented=on  Inputs=+++
  Clock : Clock  Commented=on
  Constant1 : Constant  Value=0
  Constant2 : Constant  Commented=on  Value=0
  Contratos : Subsystem
  Contribuição à Câmara : Constant  Commented=on  Value=contribuicaoCCEE
  En.Aloc - En.Cont. : Scope
      settings: SaveName=ScopeData13
  Energia alocada : Scope
      settings: SaveName=ScopeData6
  Energia contratada : Scope
      settings: SaveName=ScopeData14
  Energia Alocada : Subsystem
  Fcn{,1..3} (4 alike) : Fcn  Commented=on  Expr=u(2)*(1/(1+r)^(u(1)/52))  SampleTime=1
  Gain : Gain  Commented=on  Gain=-1
  Gain1 : Gain  Gain=-1
  Ganho com contratos : Scope
      settings: SaveName=ScopeData7
  Ganho no MRE : Scope  Commented=on
      settings: SaveName=ScopeData9
  Ganho no mercado spot : Scope
      settings: SaveName=ScopeData4
  Ganho total : Scope  Commented=on
      settings: SaveName=ScopeData12
  Geração : Subsystem  Commented=on
  Goto4 : Goto  Commented=on  GotoTag=compraMRE  TagVisibility=global
  Goto5 : Goto  Commented=on  GotoTag=vendaMRE  TagVisibility=global
  Integrator{,1..3} (4 alike) : Integrator  Commented=on
  MinMax : MinMax  Function=max  Inputs=2
  MinMax1 : MinMax  Inputs=2
  MinMax2 : MinMax  Commented=on  Function=max  Inputs=2
  MinMax3 : MinMax  Commented=on  Inputs=2
  Mux{,1..3} (4 alike) : Mux  Commented=on  Inputs=2
  PLD : Subsystem
  Product1 : Product  RndMeth=Zero
  Scope6 : Scope  Commented=on
  To Workspace : ToWorkspace  Commented=on  VariableName=Receita  SampleTime=-1  SaveFormat=Timeseries
  To Workspace2 : ToWorkspace  Commented=on  VariableName=Receita_Spot  SampleTime=-1  SaveFormat=Timeseries
  To Workspace3 : ToWorkspace  Commented=on  VariableName=Receita_Contratos  SampleTime=-1  SaveFormat=Timeseries
  To Workspace4 : ToWorkspace  Commented=on  VariableName=Receita_MRE  SampleTime=-1  SaveFormat=Timeseries
  tag scope: compraSpot=global, contratosVenda=global, vendaSpot=global
  wires:
  Mux3/1 -> Fcn3/1
  Integrator3/1 -> To Workspace4/1
  Fcn3/1 -> Integrator3/1
  Energia Alocada/1(Energia Alocada) -> Energia alocada/1, Add1/1  "em MWh"
  Contratos/1(Energia Contratada) -> Add1/2, Energia contratada/1  "em MWh"
  Geração/1(Valor MRE) -> MinMax2/2, MinMax3/2, Ganho no MRE/1
  PLD/1(PLD) -> Product1/1  "em R$/MWh"
  Product1/1 -> MinMax1/2, MinMax/2, Ganho no mercado spot/1  "em R$"
  Add1/1 -> Product1/2, En.Aloc - En.Cont./1  "em MWh"
  Integrator/1 -> To Workspace/1, Scope6/1
  Integrator1/1 -> To Workspace2/1
  Integrator2/1 -> To Workspace3/1
  Clock/1 -> Mux/1, Mux2/1, Mux3/1, Mux1/1
  Mux/1 -> Fcn/1
  Mux1/1 -> Fcn1/1
  Fcn/1 -> Integrator2/1
  Fcn1/1 -> Integrator1/1
  Fcn2/1 -> Integrator/1
  Add2/1 -> Ganho total/1, Mux2/2
  Mux2/1 -> Fcn2/1
  Constant1/1 -> MinMax1/1, MinMax/1
  Constant2/1 -> MinMax3/1, MinMax2/1
  Contratos/2(Valor Contratado) -> Ganho com contratos/1, [contratosVenda]  "em R$"
  MinMax2/1 -> Goto5/1
  MinMax3/1 -> Gain/1
  MinMax/1 -> [vendaSpot]
  MinMax1/1 -> Gain1/1
  Gain/1 -> Goto4/1
  Gain1/1 -> [compraSpot]

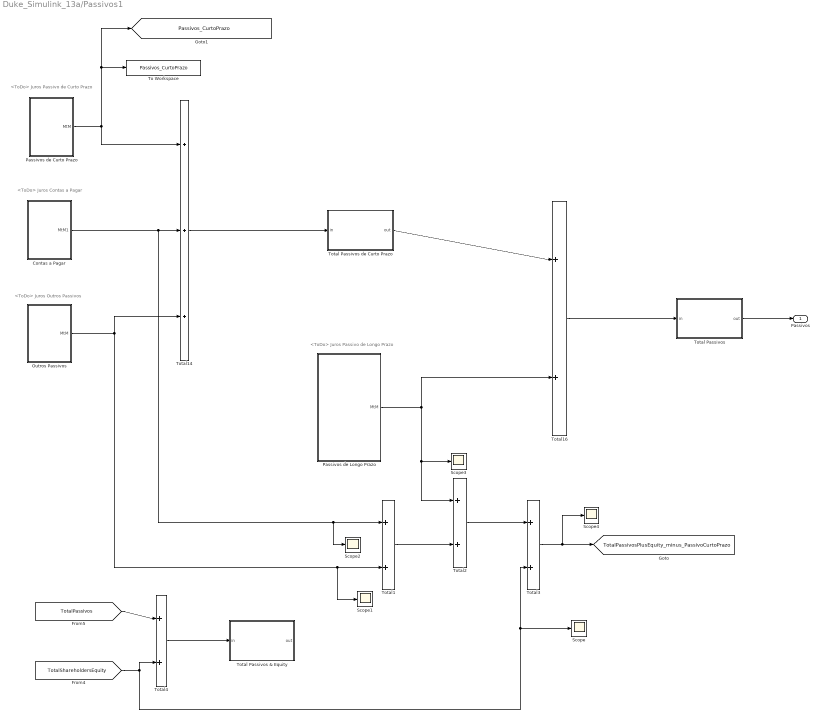
== system Duke_Simulink_13a/Passivos1 ==
  note: <ToDo>
      | Juros Passivo de Longo Prazo
  note: <ToDo>
      | Juros Outros Passivos
  note: <ToDo>
      | Juros Contas a Pagar
  note: <ToDo>
      | Juros Passivo de Curto Prazo
  Contas a Pagar : Subsystem
  Outros Passivos : Subsystem
  Passivos de Curto Prazo : Subsystem
  Passivos de Longo Prazo : Subsystem
  Scope{,1..4} (5 alike) : Scope
      Scope settings: SaveName=ScopeData77
      Scope1 settings: SaveName=ScopeData78
      Scope2 settings: SaveName=ScopeData79
      Scope3 settings: SaveName=ScopeData80
      Scope4 settings: SaveName=ScopeData97
  To Workspace : ToWorkspace  VariableName=Passivos_CurtoPrazo  SampleTime=-1  SaveFormat=Timeseries
  Total Passivos : Subsystem
  Total Passivos & Equity : Subsystem
  Total Passivos de Curto Prazo : Subsystem
  Total1 : Sum
  Total14 : Sum  Inputs=+|+|+
  Total16 : Sum  Inputs=+||+
  Total2 : Sum
  Total3 : Sum
  Total4 : Sum  Inputs=+|+
  "Passivos    " : Outport
  tag scope: Passivos_CurtoPrazo=global, TotalPassivosPlusEquity_minus_PassivoCurtoPrazo=global
  wires:
  Contas a Pagar/1(MtM1) -> Total14/2, Scope2/1, Total1/1
  Outros Passivos/1(MtM) -> Total14/3, Scope1/1, Total1/2
  Total14/1 -> Total Passivos de Curto Prazo/1(in)
  Total Passivos de Curto Prazo/1(out) -> Total16/1
  Passivos de Longo Prazo/1(MtM) -> Total2/1, Scope3/1, Total16/2
  Total16/1 -> Total Passivos/1(in)
  Passivos de Curto Prazo/1(MtM) -> [Passivos_CurtoPrazo], To Workspace/1, Total14/1
  Total Passivos/1(out) -> "Passivos    "/1
  Total4/1 -> Total Passivos & Equity/1(in)
  [TotalPassivos] -> Total4/1
  [TotalShareholdersEquity] -> Total4/2, Total3/2, Scope/1
  Total1/1 -> Total2/2
  Total2/1 -> Total3/1
  Total3/1 -> Scope4/1, [TotalPassivosPlusEquity_minus_PassivoCurtoPrazo]

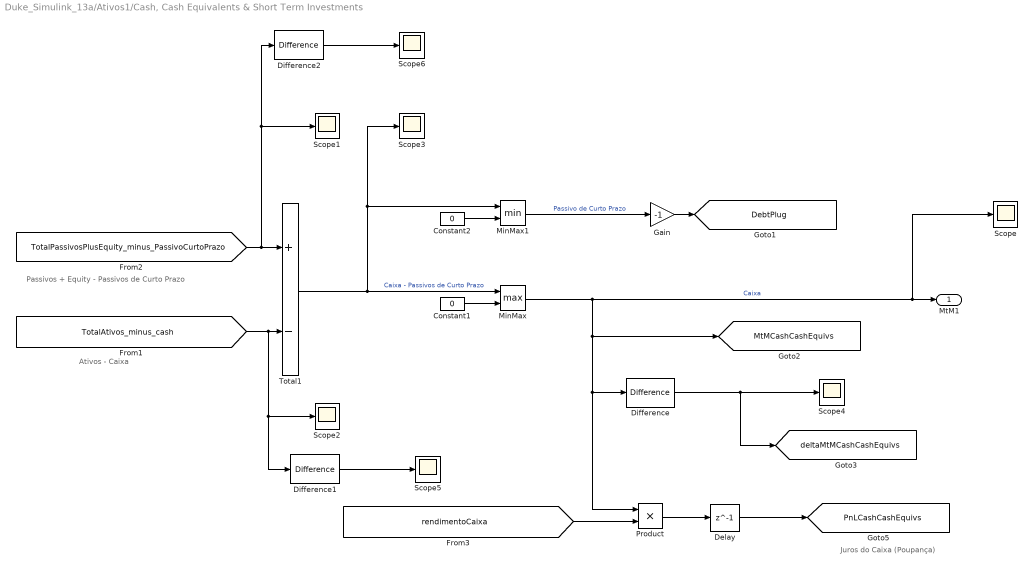
== system Duke_Simulink_13a/Ativos1/Cash, Cash Equivalents & Short Term Investments ==
  note: Juros do Caixa (Poupança)
  note: Passivos + Equity - Passivos de Curto Prazo
  note: Ativos - Caixa
  Constant1 : Constant  Value=0
  Constant2 : Constant  Value=0
  Delay : Delay  DelayLength=1  InitialCondition=0
  Difference : simulink/Discrete/Difference  ICPrevInput=CaixaInicial  InputProcessing=Inherited  OutMin=[]  OutMax=[]  OutDataType=fixdt(1, 16)  OutScaling=2^-10  DoSatur=off
  Difference1 : simulink/Discrete/Difference  ICPrevInput=0  InputProcessing=Inherited  OutMin=[]  OutMax=[]  OutDataType=fixdt(1, 16)  OutScaling=2^-10  DoSatur=off
  Difference2 : simulink/Discrete/Difference  ICPrevInput=0  InputProcessing=Inherited  OutMin=[]  OutMax=[]  OutDataType=fixdt(1, 16)  OutScaling=2^-10  DoSatur=off
  Gain : Gain  Gain=-1
  MinMax : MinMax  Function=max  Inputs=2  SampleTime=1
  MinMax1 : MinMax  Inputs=2  SampleTime=1
  Product : Product
  Scope{,1..6} (7 alike) : Scope
      Scope settings: SaveName=ScopeData19
      Scope1 settings: SaveName=ScopeData23
      Scope2 settings: SaveName=ScopeData24
      Scope3 settings: SaveName=ScopeData32
      Scope4 settings: SaveName=ScopeData51
      Scope5 settings: SaveName=ScopeData147
      Scope6 settings: SaveName=ScopeData148
  Total1 : Sum  Inputs=+-
  MtM1 : Outport
  tag scope: DebtPlug=global, MtMCashCashEquivs=global, PnLCashCashEquivs=global, deltaMtMCashCashEquivs=global
  wires:
  Total1/1 -> Scope3/1, MinMax1/1, MinMax/1  "Caixa - Passivos de Curto Prazo"
  MinMax/1 -> Scope/1, MtM1/1, Difference/1, Product/1, [MtMCashCashEquivs]  "Caixa"
  [TotalAtivos_minus_cash] -> Difference1/1, Scope2/1, Total1/2
  [TotalPassivosPlusEquity_minus_PassivoCurtoPrazo] -> Difference2/1, Scope1/1, Total1/1
  Constant1/1 -> MinMax/2
  Constant2/1 -> MinMax1/2
  MinMax1/1 -> Gain/1  "Passivo de Curto Prazo"
  Gain/1 -> [DebtPlug]
  Product/1 -> Delay/1
  [rendimentoCaixa] -> Product/2
  Delay/1 -> [PnLCashCashEquivs]
  Difference/1 -> [deltaMtMCashCashEquivs], Scope4/1
  Difference1/1 -> Scope5/1
  Difference2/1 -> Scope6/1

== system Duke_Simulink_13a/Ativos1/Contas a Receber (Recebíveis) ==
  Amostrador1 : Subsystem
  Constant : Constant  Commented=on  Value=juros_ContasAReceber
  Modified Difference : Subsystem
  Product : Product
  Sum : Sum
  MtM : Outport
  tag scope: MtMContasReceber=global, PnLContasReceber=global, PnLContasReceberCash=global, PnLContasReceberNonCash=global, deltaMtMContasReceber=global
  wires:
  Modified Difference/1(Delta) -> [deltaMtMContasReceber]
  Amostrador1/1(Out1) -> Product/1, [MtMContasReceber], MtM/1, Modified Difference/1(In1)
  ? -> Product/2
  Sum/1 -> [PnLContasReceber]

== system Duke_Simulink_13a/Ativos1/Depreciação ==
  Ativo Imobilizado Inicial : Constant  Value=PPE_Inicial
  Ativo Imobilizado Inicial2 : Constant  Value=Media_DeprPPE
  Constant2 : Constant  Value=0
  Depreciação : RandomNumber  Mean=Media_DeprPPE  Variance=Var_DeprPPE  Seed=Seed_DeprPPE
  Discrete-Time Integrator : DiscreteIntegrator  IntegratorMethod=Accumulation: Backward Euler  InitialConditionSource=external  ICPrevOutput=DiscIntNeverNeededParam  ICPrevScaledInput=DiscIntNeverNeededParam
  Product2 : Product  RndMeth=Zero
  Scope : Scope
      settings: SaveName=ScopeData71
  Scope1 : Scope
      settings: SaveName=ScopeData96
  Depreciacao : Outport
  wires:
  Ativo Imobilizado Inicial2/1 -> Product2/2
  Ativo Imobilizado Inicial/1 -> Product2/1
  Product2/1 -> Scope1/1, Discrete-Time Integrator/1
  Constant2/1 -> Discrete-Time Integrator/2
  Discrete-Time Integrator/1 -> Scope/1, Depreciacao/1

== system Duke_Simulink_13a/Ativos1/Estoque ==
  Add : Sum  Inputs=+|+|-
  Amostrador1 : Subsystem
  Modified Difference : Subsystem
  Estoque : Outport
  tag scope: Estoque=global, deltaEstoque=global
  wires:
  Modified Difference/1(Delta) -> [deltaEstoque]
  Add/1 -> [Estoque], Estoque/1, Modified Difference/1(In1)
  [ValorDoEstoqueConsolidadoDeposito] -> Amostrador1/1(In1)
  Amostrador1/1(Out1) -> Add/2

== system Duke_Simulink_13a/Ativos1/Financial Instruments (Hedging) ==
  Modified Difference1 : Subsystem
  Total11 : Sum  Inputs=+|+
  MtM : Outport
  tag scope: MtMFinInstHedge=global, PnLFinInstHedge=global, deltaMtMFinInstHedge=global
  wires:
  [PnLFinInstHedgeCash] -> Total11/1
  [PnLFinInstHedgeNonCash] -> Total11/2
  Total11/1 -> [PnLFinInstHedge]
  Modified Difference1/1(Delta) -> [deltaMtMFinInstHedge]
  [CreditoDeImposto] -> Modified Difference1/1(In1), [MtMFinInstHedge], MtM/1

== system Duke_Simulink_13a/Ativos1/Financial Instruments (Speculation) ==
  Total11 : Sum  Inputs=+|+
  MtM : Outport
  tag scope: PnLFinInstSpec=global
  wires:
  [PnLFinInstSpecCash] -> Total11/1
  [PnLFinInstSpecNonCash] -> Total11/2
  Total11/1 -> [PnLFinInstSpec]

== system Duke_Simulink_13a/Ativos1/Net PP&E ==
  Add6 : Sum  Inputs=++++++
  Add7 : Sum  Inputs=++++++
  Edificacoes : Subsystem
  Maquinas : Subsystem
  Moveis : Subsystem
  Reservatorio : Subsystem
  Scope{,1..12} (13 alike) : Scope
      Scope settings: SaveName=ScopeData54
      Scope1 settings: SaveName=ScopeData55
      Scope10 settings: SaveName=ScopeData60
      Scope11 settings: TimeRange=180  SaveName=ScopeData61
      Scope12 settings: SaveName=ScopeData146
      Scope2 settings: SaveName=ScopeData56
      Scope3 settings: SaveName=ScopeData57
      Scope4 settings: SaveName=ScopeData58
      Scope5 settings: SaveName=ScopeData59
      Scope6 settings: SaveName=ScopeData62
      Scope7 settings: SaveName=ScopeData63
      Scope8 settings: SaveName=ScopeData64
      Scope9 settings: SaveName=ScopeData65
  Terreno : Subsystem
  Veiculos : Subsystem
  Net_PP&E : Outport
  tag scope: Depreciacao_Ativos=global
  wires:
  Add6/1 -> Scope12/1, [Depreciacao_Ativos]
  Add7/1 -> Net_PP&E/1
  Reservatorio/1(Depreciacao) -> Add6/2, Scope1/1
  Edificacoes/1(Depreciacao) -> Add6/3, Scope2/1
  Maquinas/1(Depreciacao) -> Add6/4, Scope3/1
  Veiculos/1(Depreciacao) -> Add6/5, Scope4/1
  Moveis/1(Depreciacao) -> Add6/6, Scope5/1
  Terreno/2(PPE) -> Add7/1, Scope6/1
  Reservatorio/2(PPE) -> Add7/2, Scope7/1
  Edificacoes/2(PPE) -> Add7/3, Scope8/1
  Maquinas/2(PPE) -> Add7/4, Scope9/1
  Moveis/2(PPE) -> Add7/6, Scope11/1
  Veiculos/2(PPE) -> Add7/5, Scope10/1
  Terreno/1(Depreciacao) -> Add6/1

== system Duke_Simulink_13a/Ativos1/Outros Ativos ==
  Total11 : Sum  Inputs=+|+
  Outros Ativos Circulantes : Outport
  tag scope: Outros_Ativos_Circulantes=global, PnLFinInstHedge=global
  wires:
  ? -> Outros Ativos Circulantes/1, [Outros_Ativos_Circulantes]
  Total11/1 -> [PnLFinInstHedge]
  [PnLFinInstHedgeNonCash] -> Total11/2
  [PnLFinInstHedgeCash] -> Total11/1

== system Duke_Simulink_13a/Ativos1/Outros Ativos Não Circulantes ==
  out : Outport
  wires:
  ? -> out/1

== system Duke_Simulink_13a/Ativos1/Property, Plant & Equipment ==
  Amostrador2 : Subsystem
  Ativo Imobilizado Inicial : Constant  Value=PPE_Inicial
  Ativo Imobilizado Inicial1 : Constant  Value=3e6
  Investimentos : simulink/Sources/Repeating Sequence Stair  Commented=on  OutValues=Investimentos  tsamp=30  OutMin=[]  OutMax=[]  OutDataTypeStr=double  OutputDataTypeScalingMode=double  OutDataType=fixdt(0,8)  ConRadixGroup=Best Precision: Vector-wise  OutScaling=2^-12
  Product4 : Product  Commented=on  RndMeth=Zero
  Pulse Generator4 : DiscretePulseGenerator  Commented=on  Period=Periodo_Mes  PhaseDelay=DiaPgtDespesasAdm
  Total9 : Sum  Inputs=+++
  PP&E : Outport
  tag scope: InvestimentosPPE=global, NetPPE=global, deltaNetPPE=global
  wires:
  Investimentos/1 -> Product4/1
  Pulse Generator4/1 -> Product4/2
  Total9/1 -> Amostrador2/1(In1), [InvestimentosPPE]
  Product4/1 -> Total9/2
  Amostrador2/1(Out1) -> PP&E/1
  Ativo Imobilizado Inicial1/1 -> Total9/3
  [NovaUsina] -> Total9/1

== system Duke_Simulink_13a/Ativos1/Total Ativos ==
  in : Inport
  out : Outport
  tag scope: TotalAtivos=global
  wires:
  in/1 -> out/1, [TotalAtivos]

== system Duke_Simulink_13a/Ativos1/Total Ativos Operacionais ==
  in : Inport
  out : Outport
  wires:
  in/1 -> out/1

== system Duke_Simulink_13a/Ativos1/Total Ativos de Curto Prazo ==
  in : Inport
  out : Outport
  tag scope: TotalAtivosCurtoPrazo=global
  wires:
  in/1 -> [TotalAtivosCurtoPrazo], out/1

== system Duke_Simulink_13a/Equity1/Ajustes ==
  Reservatorio : Subsystem
  Ajustes : Outport
  tag scope: Ajustes=global, Depreciacao_Ajustes=global
  wires:
  Reservatorio/1(Depreciacao) -> [Depreciacao_Ajustes]
  Reservatorio/2(PPE) -> [Ajustes], Ajustes/1
